simulink library "Vehicle_Control_Axle2_Default"  (R2022b)
settings: Solver=VariableStepAuto  StartTime=0.0  StopTime=10.0  RelTol=1e-3
undefined symbols (not defined in the file): Coefficient, Pedal
libraries: Damper_Control_Axle2 x2, Brake_Control x1, Driveline_Control_Axle2_None x1, Power_Control_Axle2_FixedRatio x1, Spring_Control_Axle2 x1, Steer_Control_Axle2 x1
Description:
  | Simscape Vehicle Templates Library
  | 
  | Copyright 2018-2024 The MathWorks, Inc.
settings Model: Creator=smiller  LastModifiedBy=smiller
settings ModelReferenceCC: EnableRefExpFcnMdlSchedulingChecks=on

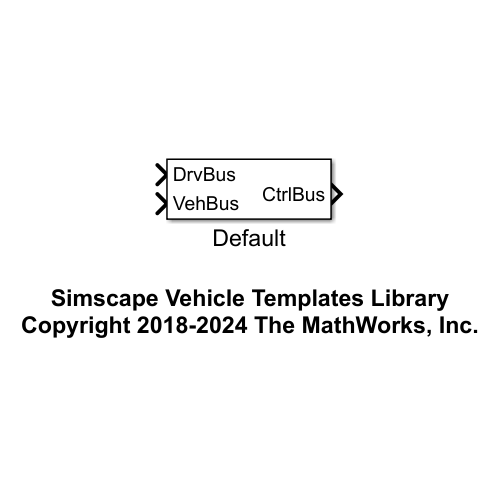
[thumbnail: Simulink's stored preview of the top-level diagram]
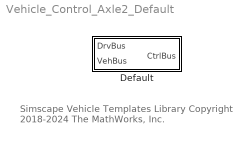
== system Vehicle_Control_Axle2_Default ==
  note: Simscape Vehicle Templates Library
      | Copyright 2018-2024 The MathWorks, Inc.
  Default : Subsystem  VariantControl=Default  mask{popup_brake_control=Pedal, popup_damper_control_A1=Coefficient, popup_damper_control_A2=Coefficient, popup_spring_control_A1=None, popup_spring_control_A2=None}
      mask prompts: popup_brake_control "Control Type"; popup_damper_control_A1 "Damper Control Axle 1"; popup_damper_control_A2 "Damper Control Axle 2"; popup_spring_control_A1 "Spring Control Axle 1"; popup_spring_control_A2 "Spring Control Axle 2"
      mask TypeOptions popup_brake_control: Brake Control/popup_brake_control
      mask TypeOptions popup_damper_control_A1: Damper Control/popup_damper_control_A1
      mask TypeOptions popup_damper_control_A2: Damper Control/popup_damper_control_A2
      mask TypeOptions popup_spring_control_A1: Spring Control/popup_spring_control_A1
      mask TypeOptions popup_spring_control_A2: Spring Control/popup_spring_control_A2

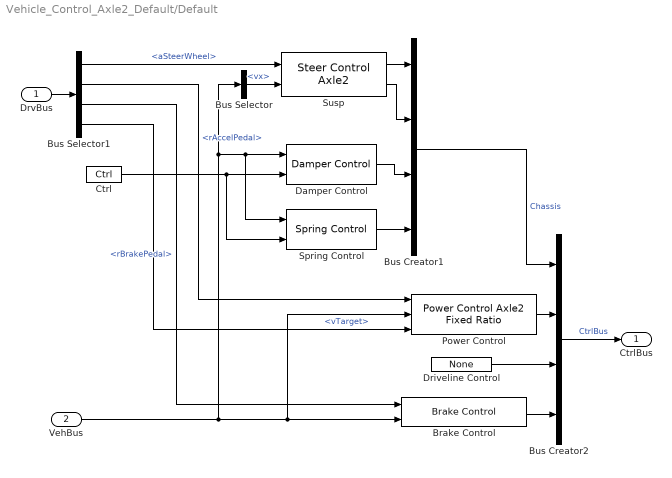
== system Vehicle_Control_Axle2_Default/Default ==
  DrvBus : Inport
  VehBus : Inport  Port=2
  Brake Control : Brake_Control/Brake Control  VariantControl=Variant1  LabelModeActiveChoice=Pedal  popup_brake_control=Pedal  abs_tire_radiusF=Vehicle.Chassis.TireA1.tire_radius.Value  abs_tire_radiusR=Vehicle.Chassis.TireA2.tire_radius.Value
      settings: AttributesFormatString=%<ActiveVariant>
  Bus Creator1 : BusCreator  Inputs=4
  Bus Creator2 : BusCreator  Inputs=4
  Bus Selector : BusSelector  OutputSignals=Chassis.Body.CG.vx
  Bus Selector1 : BusSelector  OutputSignals=aSteerWheel,rAccelPedal,rBrakePedal,Reference.vTarget
  Ctrl : Damper_Control_Axle2/Ctrl  SystemSampleTime=-1  VariantActivationTime=update diagram  Latency=0  AutoFrameSizeCalculation=off
  Damper Control : Damper_Control_Axle2/Damper Control  VariantControl=Choice  popup_damper_control_A1=Coefficient  popup_damper_control_A2=Coefficient
  Driveline Control : Driveline_Control_Axle2_None/None  SystemSampleTime=-1  VariantActivationTime=update diagram  Latency=0  AutoFrameSizeCalculation=off
  Power Control : Power_Control_Axle2_FixedRatio/Power Control Axle2 Fixed Ratio  trq_max=Control.Default.maxTrqRequest  trq_ratio_front=Control.Default.pcnt_torque_on_f  trq_rate_up=300  trq_rate_down=-5000
  Spring Control : Spring_Control_Axle2/Spring Control  VariantControl=Choice  popup_spring_control_A1=None  popup_spring_control_A2=None
  Susp : Steer_Control_Axle2/Steer Control Axle2  Steer=Control.Default.Steer
  CtrlBus : Outport  VectorParamsAs1DForOutWhenUnconnected=off
  wires:
  Bus Selector1/4 -> Power Control/3  "<vTarget>"
  Bus Selector/1 -> Susp/2  "<vx>"
  Bus Selector1/1 -> Susp/1  "<aSteerWheel>"
  Susp/2 -> Bus Creator1/2
  VehBus/1 -> Bus Selector/1, Spring Control/1, Damper Control/1, Power Control/2, Brake Control/2
  Susp/1 -> Bus Creator1/1
  Brake Control/1 -> Bus Creator2/4
  Bus Creator1/1 -> Bus Creator2/1  "Chassis"
  Damper Control/1 -> Bus Creator1/3
  Driveline Control/1 -> Bus Creator2/3
  Power Control/1 -> Bus Creator2/2
  Spring Control/1 -> Bus Creator1/4
  Bus Selector1/2 -> Power Control/1  "<rAccelPedal>"
  Bus Selector1/3 -> Brake Control/1  "<rBrakePedal>"
  Bus Creator2/1 -> CtrlBus/1  "CtrlBus"
  DrvBus/1 -> Bus Selector1/1
  Ctrl/1 -> Spring Control/2, Damper Control/2
